simulink model "LEGO_SW"  (R2019b)
settings: Solver=VariableStepAuto  StartTime=0.0  StopTime=45  RelTol=1e-3  EnableMultiTasking=on
values from neighbouring files (symbols this model uses):
  A1 = [0, 0, 1, 0;       0, 0, 0, 1;       0, -g*R*M^2*L^2/q, -2*(M*R*L + M*L^2 + Jpsi)*(Kt*Ke/Rdc + b)/q - 2*(M*L^2 + Jpsi)*b_bar/q, 2*(M*R*L + M*L^2 + Jpsi)*(Kt*Ke/Rdc + b)/q;       0, g*M*L*((2*m + M)*R^2 + 2*Jw)/q, 2*((2*m + M)*R^2 + 2*Jw + M*R*L)*(Kt*Ke/Rdc + b)/q + 2*M*R*L*b_bar/q, -2*((2*m + M)*R^2 + 2*Jw + M*R*L)*(Kt*Ke/Rdc + b)/q]    [run_LEGO_SW.m]
  A2 = [0, 1;       0, -W^2/2/R^2*(Kt*Ke/Rdc + b + b_bar)/(1/2*m*W^2 + Jphi + Jw*W^2/2/R^2)]    [run_LEGO_SW.m]
  B1 = [0; 0; 2*(M*R*L + M*L^2 + Jpsi)*Kt/Rdc/q; -2*((2*m + M)*R^2 + 2*Jw + M*R*L)*Kt/Rdc/q]    [run_LEGO_SW.m]
  B2 = [0; -W/R*Kt/Rdc/(1/2*m*W^2 + Jphi + Jw*W^2/2/R^2)]    [run_LEGO_SW.m]
  C1 = [1, 0, 0, 0;       0, 0, 0, 1]    [run_LEGO_SW.m]
  C2 = [1 0]    [run_LEGO_SW.m]
  D1 = [0;0]    [run_LEGO_SW.m]
  D2 = 0    [run_LEGO_SW.m]
  K_D_theta = -8    [run_LEGO_SW.m]
  K_P_dot_psi = -50    [run_LEGO_SW.m]
  K_P_phi = -50    [run_LEGO_SW.m]
  K_phi_OL = -A2(2,2)/B2(2)    [run_LEGO_SW.m]
  r_ID = w0^2    (= 1)    [run_LEGO_SW.m]
  r_PD = 2*xi*w0    (= 1.6)    [run_LEGO_SW.m]
  z_PI = 7    [run_LEGO_SW.m]
undefined symbols (not defined in the file or in its folder): sigbuilder_block
settings Model: SimulationMode=rapid-accelerator  Creator=KostasM  LastModifiedBy=Oskar
settings DataIOCC: LimitDataPoints=on  ReturnWorkspaceOutputs=off
settings OptimizationCC: LifeSpan=inf
settings DebuggingCC: AllowSymbolicDim=off  SFUnexpectedBacktrackingDiag=warning  SFNoUnconditionalDefaultTransitionDiag=warning  SFExecutionAtInitializationDiag=none  ArithmeticOperatorsInVariantConditions=warning
settings ModelReferenceCC: PropagateSignalLabelsOutOfModel=off
settings SFSimCC: SimUseLocalCustomCode=off  CustomCodeUndefinedFunction=UseInterfaceOnly
settings RTWCC: RTWUseLocalCustomCode=off
settings CodeAppCC: StateflowObjectComments=on
settings GRTTargetCC: TargetLangStandard=C89/C90 (ANSI)
settings ConfigComp: CovMetricSettings=dw  CovHtmlReporting=on  CovSaveCumulativeToWorkspaceVar=on  CovSaveSingleToWorkspaceVar=on  CovExternalEMLEnable=off

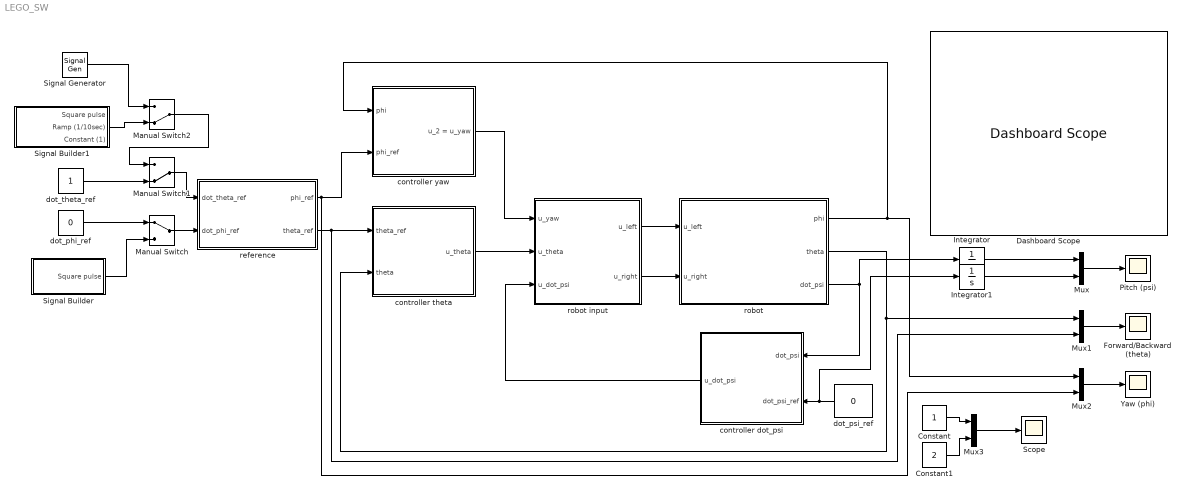
== system LEGO_SW ==
  Constant : Constant
  Constant1 : Constant  Value=2
  Dashboard Scope : DashboardScope
  Forward/Backward (theta) : Scope
  Integrator : Integrator
  Integrator1 : Integrator
  Manual Switch : ManualSwitch
  Manual Switch1 : ManualSwitch  CurrentSetting=0
  Manual Switch2 : ManualSwitch  CurrentSetting=0
  Mux{,1..3} (4 alike) : Mux  Inputs=2
  "Pitch (psi) " : Scope
  Scope : Scope
  Signal Generator : SignalGenerator  WaveForm=square  Frequency=0.1  Units=rad/sec
  Signal Builder : Subsystem  Tag=STV Subsys  LoadFcn=sigbuilder_block('load');  StartFcn=sigbuilder_block('start');  StopFcn=sigbuilder_block('stop');  ClipboardFcn=sigbuilder_block('clipboard');  mask(Sigbuilder block){tuvar=[0:10]}
      mask help: Simulink:masks:SigbuilderBlock_MD
      mask init:
      | if ~strcmp(get_param(bdroot(gcbh),'SimulationStatus'),'stopped') tuvar = sigbuilder_block('maskInit'); end
      settings: CopyFcn=sigbuilder_block('copy');  DeleteFcn=sigbuilder_block('delete');  ModelCloseFcn=sigbuilder_block('modelClose');  PreSaveFcn=sigbuilder_block('preSave');  PauseFcn=sigbuilder_block('pause');  ContinueFcn=sigbuilder_block('continue');  NameChangeFcn=sigbuilder_block('namechange');  OpenFcn=sigbuilder_block('open',[437.6 199.2 550.4 400 ]);  CloseFcn=sigbuilder_block('close');
      mask Display: plot(0, 0, 100, 100,[2, 2, 32, 32, 2], [68, 8, 8, 68, 68],[32, 2], [38, 38], [32, 19, 2],[53, 60, 44], [32, 17, 17, 2],[16, 16, 31, 31]);txt = getActiveGroup(gcbh);text(2, 100, txt,'verticalAlignment', 'top');
  Signal Builder1 : Subsystem  Tag=STV Subsys  LoadFcn=sigbuilder_block('load');  StartFcn=sigbuilder_block('start');  StopFcn=sigbuilder_block('stop');  ClipboardFcn=sigbuilder_block('clipboard');  mask(Sigbuilder block){tuvar=[0:10]}
      mask help: Simulink:masks:SigbuilderBlock_MD
      mask init:
      | if ~strcmp(get_param(bdroot(gcbh),'SimulationStatus'),'stopped') tuvar = sigbuilder_block('maskInit'); end
      settings: CopyFcn=sigbuilder_block('copy');  DeleteFcn=sigbuilder_block('delete');  ModelCloseFcn=sigbuilder_block('modelClose');  PreSaveFcn=sigbuilder_block('preSave');  PauseFcn=sigbuilder_block('pause');  ContinueFcn=sigbuilder_block('continue');  NameChangeFcn=sigbuilder_block('namechange');  OpenFcn=sigbuilder_block('open',[437.6 199.2 550.4 400 ]);  CloseFcn=sigbuilder_block('close');
      mask Display: plot(0, 0, 100, 100,[2, 2, 32, 32, 2], [68, 8, 8, 68, 68],[32, 2], [38, 38], [32, 19, 2],[53, 60, 44], [32, 17, 17, 2],[16, 16, 31, 31]);txt = getActiveGroup(gcbh);text(2, 100, txt,'verticalAlignment', 'top');
  Yaw (phi) : Scope
  controller dot_psi : Subsystem
  controller theta : Subsystem
  controller yaw : Subsystem
  "dot_phi_ref " : Constant  Value=0
  dot_psi_ref : Constant  Value=0  VectorParams1D=off
  "dot_theta_ref " : Constant
  reference : Subsystem
  robot : Subsystem
  robot input : Subsystem
  wires:
  robot/3(dot_psi) -> controller dot_psi/1("dot_psi "), Integrator/1
  robot input/1(u_left) -> robot/1(u_left)
  robot input/2(u_right) -> robot/2(u_right)
  controller theta/1(u_theta) -> robot input/2(u_theta)
  controller yaw/1(u_2 = u_yaw) -> robot input/1(u_yaw)
  reference/1(phi_ref) -> controller yaw/2(phi_ref), Mux2/2
  reference/2("theta_ref ") -> Mux1/2, controller theta/1(theta_ref)
  robot/2(theta) -> Mux1/1, controller theta/2("theta ")
  controller dot_psi/1(u_dot_psi) -> robot input/3(u_dot_psi)
  robot/1(phi) -> controller yaw/1(phi), Mux2/1
  Manual Switch/1 -> reference/2("dot_phi_ref ")
  "dot_phi_ref "/1 -> Manual Switch/1
  Mux/1 -> "Pitch (psi) "/1
  Integrator/1 -> Mux/1
  Integrator1/1 -> Mux/2
  dot_psi_ref/1 -> Integrator1/1, controller dot_psi/2(dot_psi_ref)
  Mux2/1 -> Yaw (phi)/1
  Mux1/1 -> Forward/Backward (theta)/1
  Signal Builder/1(Square pulse) -> Manual Switch/2
  Mux3/1 -> Scope/1
  Constant/1 -> Mux3/1
  Constant1/1 -> Mux3/2
  Manual Switch1/1 -> reference/1("dot_theta_ref ")
  "dot_theta_ref "/1 -> Manual Switch1/2
  Manual Switch2/1 -> Manual Switch1/1
  Signal Generator/1 -> Manual Switch2/1
  Signal Builder1/2(Ramp (1/10sec)) -> Manual Switch2/2

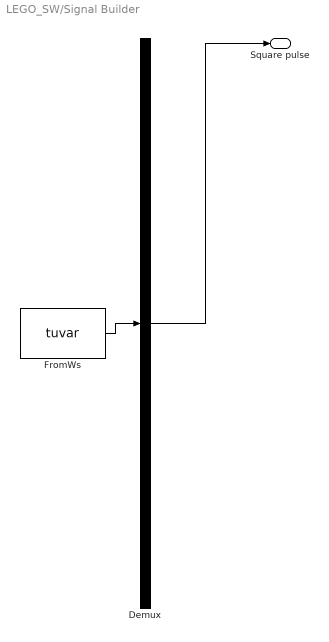
== system LEGO_SW/Signal Builder ==
  Demux : Demux  Tag=STV Demux  Outputs=1
  FromWs : FromWorkspace  Tag=STV FromWs  VariableName=tuvar  SampleTime=0
      SigBuilderData=|
      | common.afterFinalStr = 'Extrapolate'
      | common.sampleTime = 0
      | dataSet.timeRange = [0 10]
      | dataSet.name = 'Group 1'
      | sbobj.Groups.Name = 'Group 1'
      | sbobj.Groups.Signals.Name = 'Square pulse'
      | sbobj.Groups.Signals.XData = [0 4 4 6 6 10]
      | sbobj.Groups.Signals.YData = [0 0 1 1 0 0]
  Square pulse : Outport  Tag=STV Outport
  wires:
  Demux/1 -> Square pulse/1
  FromWs/1 -> Demux/1

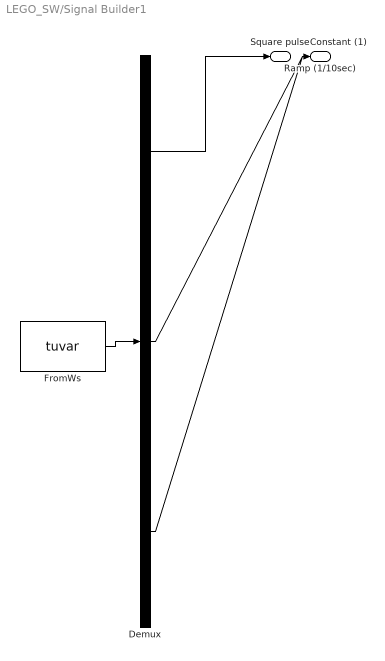
== system LEGO_SW/Signal Builder1 ==
  Demux : Demux  Tag=STV Demux  Outputs=3
  FromWs : FromWorkspace  Tag=STV FromWs  VariableName=tuvar  SampleTime=0
      SigBuilderData=|
      | common.afterFinalStr = 'Extrapolate'
      | common.sampleTime = 0
      | dataSet.timeRange = [0 10]
      | dataSet.name = 'Group 1'
      | sbobj.Groups.Name = 'Group 1'
      | sbobj.Groups.Signals(1).Name = 'Square pulse'
      | sbobj.Groups.Signals(1).XData = [0 4 4 6 6 10]
      | sbobj.Groups.Signals(1).YData = [0 0 1 1 0 0]
      | sbobj.Groups.Signals(2).Name = 'Ramp (1/10sec)'
      | sbobj.Groups.Signals(2).XData = [0 10]
      | sbobj.Groups.Signals(2).YData = [0 0.94]
      | sbobj.Groups.Signals(3).Name = 'Constant (1)'
      | sbobj.Groups.Signals(3).XData = [0 10]
      | sbobj.Groups.Signals(3).YData = [1 1]
  Square pulse : Outport  Tag=STV Outport
  Ramp (1/10sec) : Outport  Tag=STV Outport  Port=2
  Constant (1) : Outport  Tag=STV Outport  Port=3
  wires:
  Demux/1 -> Square pulse/1
  FromWs/1 -> Demux/1
  Demux/2 -> Ramp (1/10sec)/1
  Demux/3 -> Constant (1)/1

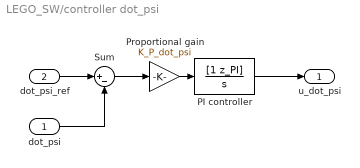
== system LEGO_SW/controller dot_psi ==
  "dot_psi " : Inport
  dot_psi_ref : Inport  Port=2
  "PI controller " : TransferFcn  Numerator=[1 z_PI]  Denominator=[1 0]
  "Proportional gain " : Gain  Gain=K_P_dot_psi
  Sum : Sum  Inputs=|+-
  u_dot_psi : Outport  VectorParamsAs1DForOutWhenUnconnected=off
  wires:
  "dot_psi "/1 -> Sum/2
  dot_psi_ref/1 -> Sum/1
  Sum/1 -> "Proportional gain "/1
  "PI controller "/1 -> u_dot_psi/1
  "Proportional gain "/1 -> "PI controller "/1

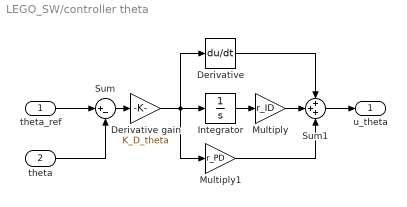
== system LEGO_SW/controller theta ==
  theta_ref : Inport
  "theta " : Inport  Port=2
  "Derivative " : Derivative  CoefficientInTFapproximation=0.00001
  "Derivative gain " : Gain  Gain=K_D_theta
  Integrator : Integrator
  Multiply : Gain  Gain=r_ID
  Multiply1 : Gain  Gain=r_PD
  Sum : Sum  Inputs=|+-
  Sum1 : Sum  Inputs=+++
  u_theta : Outport  VectorParamsAs1DForOutWhenUnconnected=off
  wires:
  theta_ref/1 -> Sum/1
  "theta "/1 -> Sum/2
  Sum/1 -> "Derivative gain "/1
  Integrator/1 -> Multiply/1
  "Derivative gain "/1 -> Multiply1/1, "Derivative "/1, Integrator/1
  Multiply/1 -> Sum1/2
  Multiply1/1 -> Sum1/3
  "Derivative "/1 -> Sum1/1
  Sum1/1 -> u_theta/1

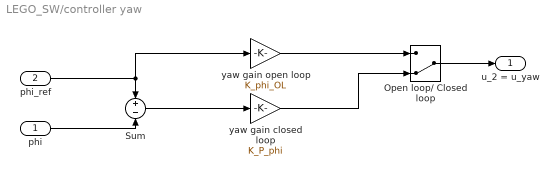
== system LEGO_SW/controller yaw ==
  phi : Inport
  phi_ref : Inport  Port=2
  "Open loop/ Closed loop " : ManualSwitch  CurrentSetting=0
  Sum : Sum  Inputs=+-
  "yaw gain closed loop " : Gain  Gain=K_P_phi
  yaw gain open loop : Gain  Gain=K_phi_OL
  u_2 = u_yaw : Outport  VectorParamsAs1DForOutWhenUnconnected=off
  wires:
  phi_ref/1 -> yaw gain open loop/1, Sum/1
  phi/1 -> Sum/2
  Sum/1 -> "yaw gain closed loop "/1
  "Open loop/ Closed loop "/1 -> u_2 = u_yaw/1
  yaw gain open loop/1 -> "Open loop/ Closed loop "/1
  "yaw gain closed loop "/1 -> "Open loop/ Closed loop "/2

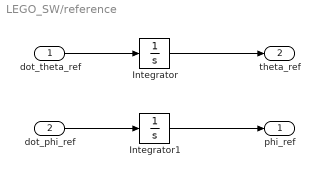
== system LEGO_SW/reference ==
  "dot_theta_ref " : Inport
  "dot_phi_ref " : Inport  Port=2
  Integrator : Integrator
  Integrator1 : Integrator
  phi_ref : Outport  VectorParamsAs1DForOutWhenUnconnected=off
  "theta_ref " : Outport  Port=2  VectorParamsAs1DForOutWhenUnconnected=off
  wires:
  "dot_theta_ref "/1 -> Integrator/1
  Integrator/1 -> "theta_ref "/1
  "dot_phi_ref "/1 -> Integrator1/1
  Integrator1/1 -> phi_ref/1

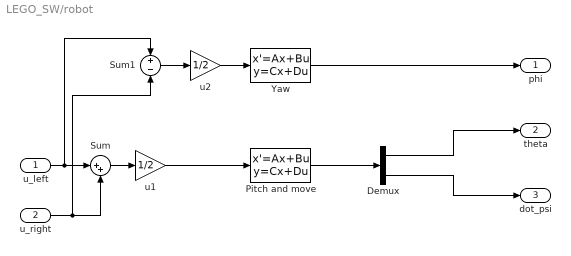
== system LEGO_SW/robot ==
  u_left : Inport
  u_right : Inport  Port=2
  Demux : Demux  Outputs=2
  "Pitch and move " : StateSpace  A=A1  B=B1  C=C1  D=D1  InitialCondition=0
  Sum : Sum  Inputs=|++
  Sum1 : Sum  Inputs=+-
  "Yaw " : StateSpace  A=A2  B=B2  C=C2  D=D2  InitialCondition=0
  "u1 " : Gain  Gain=1/2
  u2 : Gain  Gain=1/2
  phi : Outport  VectorParamsAs1DForOutWhenUnconnected=off
  theta : Outport  Port=2  VectorParamsAs1DForOutWhenUnconnected=off
  dot_psi : Outport  Port=3  VectorParamsAs1DForOutWhenUnconnected=off
  wires:
  u_left/1 -> Sum1/1, Sum/1
  u_right/1 -> Sum1/2, Sum/2
  Sum/1 -> "u1 "/1
  "u1 "/1 -> "Pitch and move "/1
  "Pitch and move "/1 -> Demux/1
  Demux/1 -> theta/1
  Demux/2 -> dot_psi/1
  "Yaw "/1 -> phi/1
  u2/1 -> "Yaw "/1
  Sum1/1 -> u2/1

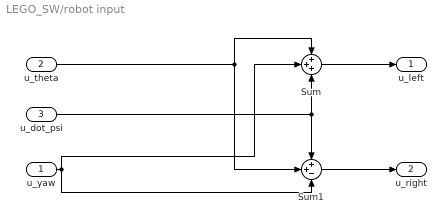
== system LEGO_SW/robot input ==
  u_yaw : Inport
  u_theta : Inport  Port=2
  u_dot_psi : Inport  Port=3
  Sum : Sum  Inputs=+++
  Sum1 : Sum  Inputs=++-
  u_left : Outport  VectorParamsAs1DForOutWhenUnconnected=off
  u_right : Outport  Port=2  VectorParamsAs1DForOutWhenUnconnected=off
  wires:
  u_theta/1 -> Sum/1, Sum1/2
  u_dot_psi/1 -> Sum/3, Sum1/1
  Sum/1 -> u_left/1
  Sum1/1 -> u_right/1
  u_yaw/1 -> Sum1/3, Sum/2
